simulink model "wAOORandVOOR"  (R2023b)
settings: Solver=FixedStepAuto  StartTime=0.0  StopTime=10.0  FixedStep=1e-3  RelTol=1e-3  EnableMultiTasking=on
undefined symbols (not defined in the file or in its folder): A0, D0, D1, D10, D11, D12, D13, D2, D3, D4, D5, D6, D7, D8, D9, PTA0, PTA1, PTA2, PTB2, PTB23, PTB9, PTC16, PTC17, PTC2, PTC3, PTC4, PTD0, PTD1, PTD2, PTD3
libraries: frdmk64flib x17
settings Model: ExtModeTrigDuration=5  Creator=emily  LastModifiedBy=nabih
settings SolverCC: AlgebraicLoopSolver=TrustRegion
settings OptimizationCC: EnhancedBackFolding=on  PassReuseOutputArgsAs=Individual arguments  ZeroExternalMemoryAtStartup=off  ZeroInternalMemoryAtStartup=off  MaxStackSize=64  OptimizeBlockOrder=speed  DifferentSizesBufferReuse=on  OptimizationCustomize=off  EfficientTunableParamExpr=on
settings DebuggingCC: ParameterTunabilityLossMsg=error  UnconnectedInputMsg=warning  UnconnectedOutputMsg=warning  UnconnectedLineMsg=warning
settings HardwareCC: ProdBitPerPointer=32  ProdBitPerSizeT=32  ProdBitPerPtrDiffT=32  ProdLargestAtomicInteger=Long  ProdLargestAtomicFloat=Double  ProdWordSize=32  ProdHWDeviceType=ARM Compatible->ARM Cortex
settings ModelReferenceCC: EnableRefExpFcnMdlSchedulingChecks=on
settings SFSimCC: MATLABDynamicMemAlloc=off
settings RTWCC: Description=Embedded Coder  SystemTargetFile=ert.tlc  HardwareBoard=NXP FRDM-K64F  TLCOptions="-aInlineSetEventsForThisBaseRateFcn=TLC_FALSE -aSuppressMultiTaskScheduler=TLC_FALSE  -aRateBasedStepFcn=0"  TemplateMakefile=ert_default_tmf  Toolchain=GNU Tools for ARM Embedded Processors
settings CodeAppCC: ForceParamTrailComments=on  IgnoreCustomStorageClasses=off  OperatorAnnotations=on  SimulinkDataObjDesc=on  SFDataObjDesc=on  InsertBlockDesc=on

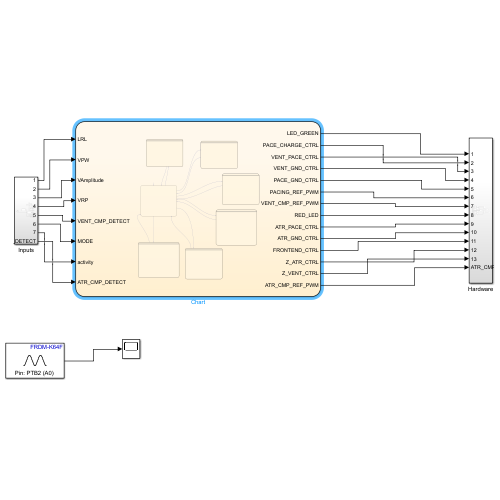
[thumbnail: Simulink's stored preview of the top-level diagram]
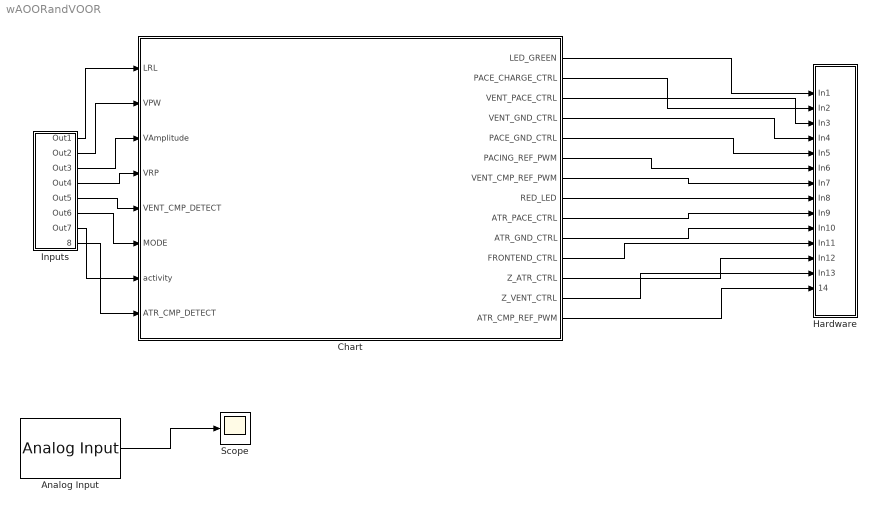
== system wAOORandVOOR ==
  Analog Input : frdmk64flib/Analog Input  Whichpin=PTB2 (A0)  SampleTime=-1
  Chart : Stateflow chart  TreatAsAtomicUnit=on
  Hardware : Subsystem
  Inputs : Subsystem
  Scope : Scope
  wires:
  Chart/2(PACE_CHARGE_CTRL) -> Hardware/2(In2)
  Chart/4(VENT_GND_CTRL) -> Hardware/4(In4)
  Chart/12(Z_ATR_CTRL) -> Hardware/12(In12)
  Inputs/4(Out4) -> Chart/4(VRP)
  Chart/7(VENT_CMP_REF_PWM) -> Hardware/7(In7)
  Inputs/5(Out5) -> Chart/5(VENT_CMP_DETECT)
  Inputs/3(Out3) -> Chart/3(VAmplitude)
  Chart/3(VENT_PACE_CTRL) -> Hardware/3(In3)
  Inputs/6(Out6) -> Chart/6(MODE)
  Inputs/1(Out1) -> Chart/1(LRL)
  Chart/6(PACING_REF_PWM) -> Hardware/6(In6)
  Chart/13(Z_VENT_CTRL) -> Hardware/13(In13)
  Chart/9(ATR_PACE_CTRL) -> Hardware/9(In9)
  Chart/11(FRONTEND_CTRL) -> Hardware/11(In11)
  Chart/8(RED_LED) -> Hardware/8(In8)
  Chart/10(ATR_GND_CTRL) -> Hardware/10(In10)
  Inputs/2(Out2) -> Chart/2(VPW)
  Chart/5(PACE_GND_CTRL) -> Hardware/5(In5)
  Chart/1(LED_GREEN) -> Hardware/1(In1)
  Inputs/7(Out7) -> Chart/7(activity)
  Inputs/8(ATR_CMP_DETECT) -> Chart/8(ATR_CMP_DETECT)
  Chart/14(ATR_CMP_REF_PWM) -> Hardware/14(ATR_CMP_REF_PWM)
  Analog Input/1 -> Scope/1

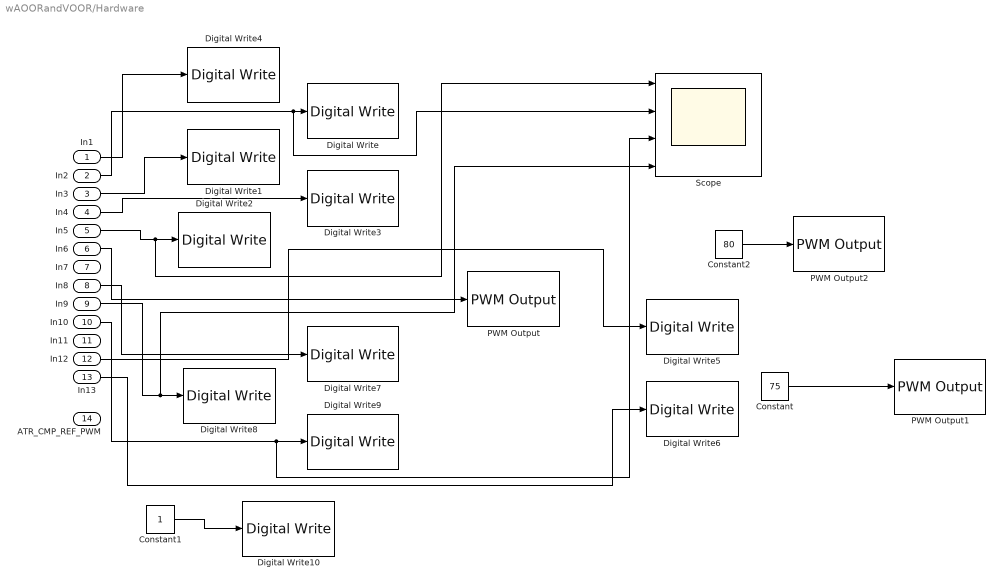
== system wAOORandVOOR/Hardware ==
  In1 : Inport
  In2 : Inport  Port=2
  In3 : Inport  Port=3
  In4 : Inport  Port=4
  In5 : Inport  Port=5
  In6 : Inport  Port=6
  In7 : Inport  Port=7
  In8 : Inport  Port=8
  In9 : Inport  Port=9
  In10 : Inport  Port=10
  In11 : Inport  Port=11
  In12 : Inport  Port=12
  In13 : Inport  Port=13
  ATR_CMP_REF_PWM : Inport  Port=14
  Constant : Constant  Value=75
  Constant1 : Constant
  Constant2 : Constant  Value=80
  Digital Write : frdmk64flib/Digital Write  Whichpin=PTB9 (D2)
  Digital Write1 : frdmk64flib/Digital Write  Whichpin=PTC4 (D9)
  Digital Write10 : frdmk64flib/Digital Write  Whichpin=PTD1 (D13)
  Digital Write2 : frdmk64flib/Digital Write  Whichpin=PTD0 (D10)
  Digital Write3 : frdmk64flib/Digital Write  Whichpin=PTD3 (D12)
  Digital Write4 : frdmk64flib/Digital Write  Whichpin=GREEN_LED
  Digital Write5 : frdmk64flib/Digital Write  Whichpin=PTB23 (D4)
  Digital Write6 : frdmk64flib/Digital Write  Whichpin=PTC3 (D7)
  Digital Write7 : frdmk64flib/Digital Write  Whichpin=RED_LED
  Digital Write8 : frdmk64flib/Digital Write  Whichpin=PTA0 (D8)
  Digital Write9 : frdmk64flib/Digital Write  Whichpin=PTD2 (D11)
  PWM Output : frdmk64flib/PWM Output  Whichpin=PTA2 (D5)  InitialFrequency=2000  InitialDutyCycle=30
  PWM Output1 : frdmk64flib/PWM Output  Whichpin=PTA1 (D3)  InitialFrequency=2000  InitialDutyCycle=0
  PWM Output2 : frdmk64flib/PWM Output  Whichpin=PTC2 (D6)  InitialFrequency=2000  InitialDutyCycle=0
  Scope : Scope  NumInputPorts=4
  wires:
  In10/1 -> Scope/3, Digital Write9/1
  In2/1 -> Scope/2, Digital Write/1
  In6/1 -> PWM Output/1
  In4/1 -> Digital Write3/1
  In13/1 -> Digital Write6/1
  In1/1 -> Digital Write4/1
  In5/1 -> Scope/1, Digital Write2/1
  In3/1 -> Digital Write1/1
  In9/1 -> Scope/4, Digital Write8/1
  In8/1 -> Digital Write7/1
  In12/1 -> Digital Write5/1
  Constant/1 -> PWM Output1/1
  Constant1/1 -> Digital Write10/1
  Constant2/1 -> PWM Output2/1

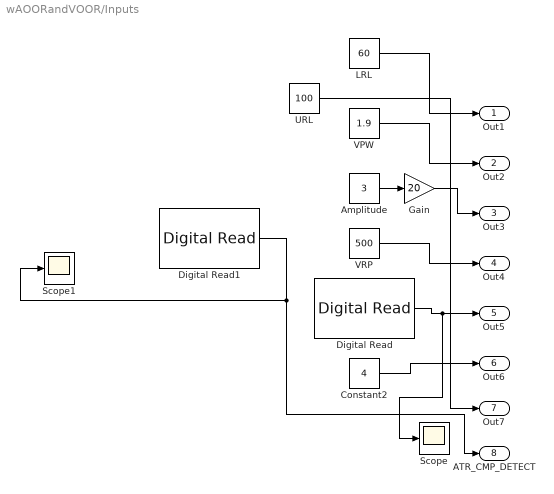
== system wAOORandVOOR/Inputs ==
  Amplitude : Constant  Value=3
  Constant2 : Constant  Value=4  OutDataTypeStr=int16
  Digital Read : frdmk64flib/Digital Read  Whichpin=PTC17 (D1)  SampleTime=inf
  Digital Read1 : frdmk64flib/Digital Read  Whichpin=PTC16 (D0)  SampleTime=-1
  Gain : Gain  Gain=20
  LRL : Constant  Value=60
  Scope : Scope
  Scope1 : Scope
  URL : Constant  Value=100
  VPW : Constant  Value=1.9  OutDataTypeStr=double
  VRP : Constant  Value=500
  Out1 : Outport
  Out2 : Outport  Port=2
  Out3 : Outport  Port=3
  Out4 : Outport  Port=4
  Out5 : Outport  Port=5
  Out6 : Outport  Port=6
  Out7 : Outport  Port=7
  ATR_CMP_DETECT : Outport  Port=8
  wires:
  VPW/1 -> Out2/1
  Amplitude/1 -> Gain/1
  Digital Read/1 -> Out5/1, Scope/1
  VRP/1 -> Out4/1
  Constant2/1 -> Out6/1
  LRL/1 -> Out1/1
  Gain/1 -> Out3/1
  URL/1 -> Out7/1
  Digital Read1/1 -> Scope1/1, ATR_CMP_DETECT/1

== stateflow chart wAOORandVOOR/Chart ==
  state AOOR
    entry:
    PACE_GND_CTRL  = 1;
    PACING_REF_PWM = VAmplitude;
    current_rate = LRL;
    interval_ms  = 60000 / current_rate;
    state TIMING
      entry:
      LED_GREEN = 0;
      ATR_PACE_CTRL = 0;
      PACE_CHARGE_CTRL =1;
      ATR_GND_CTRL = 1;
      entry:
      LED_GREEN      = 0;
      ATR_PACE_CTRL  = 0;
      PACE_CHARGE_CTRL = 1;
      ATR_GND_CTRL   = 1;
      during:
      % map activity to a rate between LRL and MAX_RATE
      current_rate = LRL + activity * (MAX_RATE - LRL);
      % clamp to valid range
      if current_rate < LRL
      current_rate = LRL;
      elseif current_rate > MAX_RATE
      current_rate = MAX_RATE;
      end
      % compute interval in ms
      interval_ms = 60000 / current_rate;
    state PULSE
      entry:
      LED_GREEN = 1;
      PACE_CHARGE_CTRL =0;
      ATR_GND_CTRL = 0;
      ATR_PACE_CTRL = 1;
    (default) -> AOOR.TIMING
    AOOR.TIMING -> AOOR.PULSE : after(interval_ms - VPW, msec)
    AOOR.PULSE -> AOOR.TIMING : after(VPW, msec)
  state AOO
    entry:
    PACE_GND_CTRL = 1;
    PACING_REF_PWM = VAmplitude;
    state TIMING
      entry:
      LED_GREEN = 0;
      ATR_PACE_CTRL = 0;
      PACE_CHARGE_CTRL =1;
      ATR_GND_CTRL = 1;
    state PULSE
      entry:
      LED_GREEN = 1;
      PACE_CHARGE_CTRL =0;
      ATR_GND_CTRL = 0;
      ATR_PACE_CTRL = 1;
    (default) -> AOO.TIMING
    AOO.PULSE -> AOO.TIMING : after(VPW, msec)
    AOO.TIMING -> AOO.PULSE : after(60000/LRL -VPW, msec)
  state VOO
    entry:
    PACE_GND_CTRL = 1;
    PACING_REF_PWM = VAmplitude;
    state TIMING
      entry:
      LED_GREEN = 0;
      VENT_PACE_CTRL = 0;
      PACE_CHARGE_CTRL =1;
      VENT_GND_CTRL = 1;
    state PULSE
      entry:
      LED_GREEN = 1;
      PACE_CHARGE_CTRL =0;
      VENT_PACE_CTRL = 1;
      VENT_GND_CTRL = 0;
    (default) -> VOO.TIMING
    VOO.PULSE -> VOO.TIMING : after(VPW, msec)
    VOO.TIMING -> VOO.PULSE : after(60000/LRL -VPW, msec)
  state INITIALIZE
    entry:
    PACE_CHARGE_CTRL = 0;
    ATR_PACE_CTRL = 0;
    VENT_PACE_CTRL = 0;
    PACE_GND_CTRL = 1;
    ATR_GND_CTRL = 0;
    VENT_GND_CTRL=0;
    FRONTEND_CTRL=1;
    Z_ATR_CTRL = 0;
    Z_VENT_CTRL=0;
  state VVI
    entry:
    PACE_GND_CTRL = 1;
    PACING_REF_PWM = VAmplitude;
    VENT_CMP_REF_PWM=60;
    FRONTEND_CTRL = 1;
    state WAIT
      entry:
      FRONTEND_CTRL = 1;
      PACE_CHARGE_CTRL = 1;
      Z_VENT_CTRL=1;
      VENT_PACE_CTRL = 0;
      VENT_GND_CTRL =1;
      RED_LED = 0;
      LED_GREEN = 0;
    state PACE
      entry:
      PACE_CHARGE_CTRL = 0;
      Z_VENT_CTRL=0;
      VENT_PACE_CTRL = 1;
      VENT_GND_CTRL = 0;
      RED_LED = 0;
      LED_GREEN = 1;
    state REFRACTORY
      entry:
      FRONTEND_CTRL=0;
      PACE_CHARGE_CTRL = 1;
      Z_VENT_CTRL=1;
      VENT_PACE_CTRL = 0;
      VENT_GND_CTRL = 1;
      RED_LED = 1;
      LED_GREEN = 0;
    (default) -> VVI.WAIT
    VVI.WAIT -> VVI.PACE [order 1] : after(60000/LRL -VPW, msec)
    VVI.WAIT -> VVI.REFRACTORY [order 2] : [VENT_CMP_DETECT==1]
    VVI.REFRACTORY -> VVI.WAIT : after(VRP, msec)
    VVI.PACE -> VVI.REFRACTORY : after(VPW,msec)
  state AAI
    entry:
    PACE_GND_CTRL = 1;
    PACING_REF_PWM = VAmplitude;
    FRONTEND_CTRL = 1;
    ATR_CMP_REF_PWM=60;
    state PACE
      entry:
      PACE_CHARGE_CTRL = 0;
      ATR_PACE_CTRL = 1;
      ATR_GND_CTRL = 0;
      RED_LED = 0;
      LED_GREEN = 1;
    state WAIT
      entry:
      FRONTEND_CTRL = 1;
      PACE_CHARGE_CTRL = 1;
      ATR_PACE_CTRL = 0;
      ATR_GND_CTRL =1;
      RED_LED = 0;
      LED_GREEN = 0;
    state REFRACTORY
      entry:
      FRONTEND_CTRL=0;
      PACE_CHARGE_CTRL = 1;
      ATR_PACE_CTRL = 0;
      ATR_GND_CTRL = 1;
      RED_LED = 1;
      LED_GREEN = 0;
    (default) -> AAI.WAIT
    AAI.WAIT -> AAI.PACE [order 1] : after(60000/LRL -VPW, msec)
    AAI.WAIT -> AAI.REFRACTORY [order 2] : [ATR_CMP_DETECT==1]
    AAI.REFRACTORY -> AAI.WAIT : after(VRP, msec)
    AAI.PACE -> AAI.REFRACTORY : after(VPW,msec)
  state VOOR
    entry:
    PACE_GND_CTRL  = 1;
    PACING_REF_PWM = VAmplitude;
    current_rate   = LRL;
    interval_ms    = 60000 / current_rate;
    state TIMING
      entry:
      LED_GREEN = 0;
      VENT_PACE_CTRL = 0;
      PACE_CHARGE_CTRL =1;
      VENT_GND_CTRL = 1;
      during:
      % map activity to a rate between LRL and MAX_RATE
      current_rate = LRL + activity * (MAX_RATE - LRL);
      % clamp to valid range
      if current_rate < LRL
      current_rate = LRL;
      elseif current_rate > MAX_RATE
      current_rate = MAX_RATE;
      end
      % compute interval in ms
      interval_ms = 60000 / current_rate;
    state PULSE
      entry:
      LED_GREEN = 1;
      PACE_CHARGE_CTRL =0;
      VENT_PACE_CTRL = 1;
      VENT_GND_CTRL = 0;
    (default) -> VOOR.TIMING
    VOOR.TIMING -> VOOR.PULSE : after(interval_ms - VPW, msec)
    VOOR.PULSE -> VOOR.TIMING : after(VPW, msec)
  INITIALIZE -> AOO [order 1] : [MODE==1]
  AOO -> INITIALIZE : [MODE~=1]
  AOOR -> INITIALIZE : [MODE==~5]
  INITIALIZE -> AOOR [order 5] : [MODE==5]
  INITIALIZE -> VOO [order 2] : [MODE==2]
  (default) -> INITIALIZE
  VOO -> INITIALIZE : [MODE~=2]
  INITIALIZE -> VVI [order 4] : [MODE==3]
  VVI -> INITIALIZE : [MODE~=3]
  INITIALIZE -> VOOR [order 6] : [MODE==6]
  AAI -> INITIALIZE : [MODE~=4]
  INITIALIZE -> AAI [order 3] : [MODE==4]
  VOOR -> INITIALIZE : [MODE==~6]
  data: LRL input; VPW input double; LED_GREEN output int16; PACE_CHARGE_CTRL output int16; VENT_PACE_CTRL output int16; VENT_GND_CTRL output int16; PACE_GND_CTRL output int16; PACING_REF_PWM output double; VAmplitude input double; VRP input; VENT_CMP_DETECT input boolean; MODE input int16; VENT_CMP_REF_PWM output; RED_LED output; ATR_PACE_CTRL output; ATR_GND_CTRL output; FRONTEND_CTRL output; Z_ATR_CTRL output; Z_VENT_CTRL output; activity input; ATR_CMP_DETECT input; ATR_CMP_REF_PWM output; current_rate local; interval_ms local; MAX_RATE local =120
